simulink model "IGVC2023_LaneLines_PublishingwLabels"  (R2022a)
settings: Solver=FixedStepAuto  StartTime=0.0  StopTime=inf  RelTol=1e-3  AbsTol=1e-3
model workspace (MAT data in the model file):
  SL_ROS_VariableLengthArrays_MaxSizes.CommonInfo.ArrayTruncateAction = 'EmitWarning'
  SL_ROS_VariableLengthArrays_MaxSizes.MsgTypeMap = containers.Map
  SL_ROS_VariableLengthArrays_MaxSizes.MsgTypeMap.serialization.keys = {'sensor_msgs/Image', 'sensor_msgs/PointCloud2'}
  SL_ROS_VariableLengthArrays_MaxSizes.MsgTypeMap.serialization.values{1}(1).PropertyName = 'Data'
  SL_ROS_VariableLengthArrays_MaxSizes.MsgTypeMap.serialization.values{1}(1).DataType = 'uint8'
  SL_ROS_VariableLengthArrays_MaxSizes.MsgTypeMap.serialization.values{1}(1).MaxLength = 3686400
  SL_ROS_VariableLengthArrays_MaxSizes.MsgTypeMap.serialization.values{1}(2).PropertyName = 'Encoding'
  SL_ROS_VariableLengthArrays_MaxSizes.MsgTypeMap.serialization.values{1}(2).DataType = 'uint8'
  SL_ROS_VariableLengthArrays_MaxSizes.MsgTypeMap.serialization.values{1}(2).MaxLength = 128
  SL_ROS_VariableLengthArrays_MaxSizes.MsgTypeMap.serialization.values{2}(1).PropertyName = 'Data'
  SL_ROS_VariableLengthArrays_MaxSizes.MsgTypeMap.serialization.values{2}(1).DataType = 'uint8'
  SL_ROS_VariableLengthArrays_MaxSizes.MsgTypeMap.serialization.values{2}(1).MaxLength = 100000
  SL_ROS_VariableLengthArrays_MaxSizes.MsgTypeMap.serialization.values{2}(2).PropertyName = 'Fields'
  SL_ROS_VariableLengthArrays_MaxSizes.MsgTypeMap.serialization.values{2}(2).DataType = 'sensor_msgs/PointField'
  SL_ROS_VariableLengthArrays_MaxSizes.MsgTypeMap.serialization.values{2}(2).MaxLength = 16
  SL_ROS_VariableLengthArrays_MaxSizes.MsgTypeMap.serialization.uniformity = 0
  SL_ROS_VariableLengthArrays_MaxSizes.MsgTypeMap.serialization.keyType = 'char'
  SL_ROS_VariableLengthArrays_MaxSizes.MsgTypeMap.serialization.valueType = 'any'
undefined symbols (not defined in the file): coder, gray, ros
libraries: robotlib x42, visionconversions x2, visionmorphops x2, visiongeotforms x2, visionstatistics x1, visionsources x1
settings Model: Creator=ll  LastModifiedBy=ll
settings OptimizationCC: EnhancedBackFolding=on  PassReuseOutputArgsAs=Individual arguments  ZeroExternalMemoryAtStartup=off  ZeroInternalMemoryAtStartup=off  MaxStackSize=64  OptimizeBlockOrder=speed  DifferentSizesBufferReuse=on  OptimizationCustomize=off  EfficientTunableParamExpr=on
settings DebuggingCC: ParameterTunabilityLossMsg=error
settings HardwareCC: ProdBitPerPointer=32  ProdBitPerSizeT=32  ProdBitPerPtrDiffT=32  ProdLargestAtomicFloat=None  ProdIntDivRoundTo=Undefined  ProdEndianess=Unspecified  ProdWordSize=32  ProdHWDeviceType=Generic->Unspecified (assume 32-bit Generic)
settings RTWCC: SystemTargetFile=ert.tlc  HardwareBoard=Robot Operating System (ROS)  TLCOptions="-aInlineSetEventsForThisBaseRateFcn=TLC_FALSE -aSuppressMultiTaskScheduler=TLC_FALSE  -aRateBasedStepFcn=0"  TemplateMakefile=ert_default_tmf  Toolchain=Catkin  TargetLang=C++
settings CodeAppCC: ForceParamTrailComments=on  IgnoreCustomStorageClasses=off  OperatorAnnotations=on  SimulinkDataObjDesc=on  SFDataObjDesc=on  InsertBlockDesc=on
settings ERTTargetCC: SupportVariableSizeSignals=on

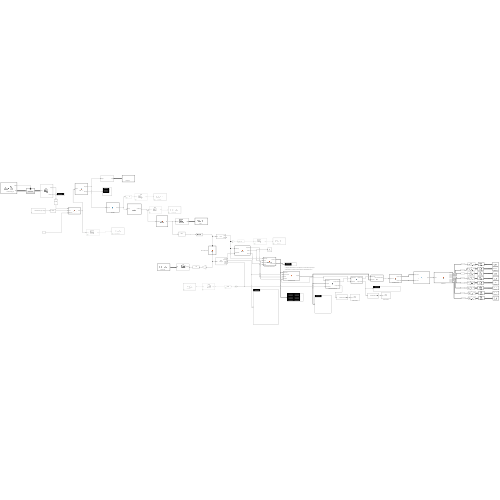
[thumbnail: Simulink's stored preview of the top-level diagram]
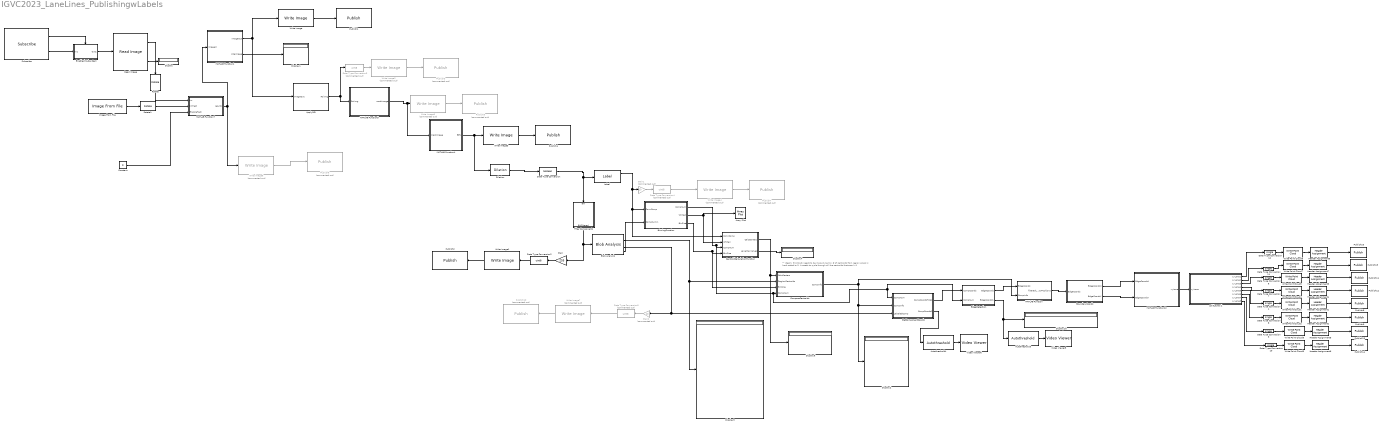
== system IGVC2023_LaneLines_PublishingwLabels ==
  note: ** ideally this block needs to be more dynamic, # of centroids from region props
      | is hard coded to 3. it needs to cycle through all the centroids that aren't -1
  ApplyROI : MATLAB Function  TreatAsAtomicUnit=on
  Array Plot : ArrayPlot  WindowPosition=[1055.000000,29.000000,800.000000,500.000000,]  ScopeFrameLocation=window  MaximizeAxes=Off
  Autothreshold3 : visionconversions/Autothreshold  operator=>  threshOut=off  effMetricOut=off  userDefinedRange=off  umin=0  umax=255  outOfRngOpt=Ignore  scaleThreshold=off  scaleFactor=1  roundingMode=Floor  overflowMode=off  P1Mode=Specify word length  P1WordLength=32  P1FracLength=30  P2Mode=Specify word length  P2WordLength=32  P2FracLength=22  P3Mode=Specify word length  P3WordLength=32  P3FracLength=14  P4Mode=Binary point scaling  P4WordLength=32  P4FracLength=15  Q1Mode=Specify word length  Q1WordLength=32  Q1FracLength=16  EMMode=Specify word length  EMWordLength=16  EMFracLength=14
      settings: SourceProductBaseCode=VP
  Autothreshold4 : visionconversions/Autothreshold  operator=>  threshOut=off  effMetricOut=off  userDefinedRange=off  umin=0  umax=255  outOfRngOpt=Ignore  scaleThreshold=off  scaleFactor=1  roundingMode=Floor  overflowMode=off  P1Mode=Specify word length  P1WordLength=32  P1FracLength=30  P2Mode=Specify word length  P2WordLength=32  P2FracLength=22  P3Mode=Specify word length  P3WordLength=32  P3FracLength=14  P4Mode=Binary point scaling  P4WordLength=32  P4FracLength=15  Q1Mode=Specify word length  Q1WordLength=32  Q1FracLength=16  EMMode=Specify word length  EMWordLength=16  EMFracLength=14
      settings: SourceProductBaseCode=VP
  BinningFunction : MATLAB Function  TreatAsAtomicUnit=on
  Blob Analysis : visionstatistics/Blob Analysis  Tag=vipblks_row_conv  area=on  centroid=on  bBox=on  majorAxis=off  minorAxis=off  angle=off  eccentricity=off  equivDiameterSq=off  extent=off  perimeter=off  outDT=double  conn=8  isLabel=on  maxBlobs=10000  warnIfNumBlobsExceeded=on  isCount=on  useMinArea=off  minArea=0  useMaxArea=off  maxArea=intmax('uint32')  excludeBorderBlob=off  isOutVarDim=off  isFill=on  fillValues=-1  roundingMode=Floor  overflowMode=off  prodOutputMode=Binary point scaling  prodOutputWordLength=32  prodOutputFracLength=16  accumMode=Binary point scaling  accumWordLength=32  accumFracLength=0  outputMode=Binary point scaling  outputWordLength=32  outputFracLength=16  firstCoeffMode=Binary point scaling  firstCoeffWordLength=16  firstCoeffFracLength=14  secondCoeffMode=Binary point scaling  secondCoeffWordLength=32  secondCoeffFracLength=16
  BoundaryCoords : MATLAB Function  TreatAsAtomicUnit=on
  CentroidCalculationFunction : MATLAB Function  TreatAsAtomicUnit=on
  CompareCentroids : MATLAB Function  TreatAsAtomicUnit=on
  Constant : Constant  Value=0
  Data Type Conversion : DataTypeConversion  OutDataTypeStr=boolean  SaturateOnIntegerOverflow=off  RndMeth=Floor
  Data Type Conversion{1,6..12} (8 alike) : DataTypeConversion  OutDataTypeStr=single  SaturateOnIntegerOverflow=off  RndMeth=Floor
  Data Type Conversion2 : DataTypeConversion  OutDataTypeStr=uint8  SaturateOnIntegerOverflow=off  RndMeth=Floor
  Data Type Conversion3 : DataTypeConversion  Commented=on  OutDataTypeStr=uint8  SaturateOnIntegerOverflow=off  RndMeth=Floor
  Data Type Conversion4 : DataTypeConversion  Commented=on  OutDataTypeStr=uint8  SaturateOnIntegerOverflow=off  RndMeth=Floor
  Data Type Conversion5 : DataTypeConversion  Commented=on  OutDataTypeStr=uint8  SaturateOnIntegerOverflow=off  RndMeth=Floor
  Dilation : visionmorphops/Dilation  nhoodsrc=Specify via dialog  strel=[1 1 1; 1 1 1; 1 1 1]
      settings: SourceProductBaseCode=VP
  Display{,1..4,6,16} (7 alike) : Display
  EdgeDetection : MATLAB Function  TreatAsAtomicUnit=on
  Enabled Subsystem : Subsystem  TreatAsAtomicUnit=on
  "Filter Components " : MATLAB Function  TreatAsAtomicUnit=on
  Gain : Gain  Gain=255
  Gain1 : Gain  Commented=on  Gain=10
  Gain2 : Gain  Commented=on  Gain=10
  GetComponentCoords : MATLAB Function  TreatAsAtomicUnit=on
  Header Assignment{1..8} (8 alike) : robotlib/Header Assignment  SetFrameID=on  FrameID=map  InsertTimeStamp=on  SetHeaderFieldName=Use the default Header field name  HeaderFieldName=Header
      settings: SourceProductBaseCode=RR
  Image From File : visionsources/Image From File  Tag=vipblks_nd  FileName=/home/ll/catkin_ws/lanesonCourse.png  Ts=inf  imagePorts=One multidimensional signal  OutPortLabels=R|G|B  ImageDataType=Inherit from input image  sdImageDataType=uint(8)  Signed=on  WordLength=16  FractionLengthMode=User-defined  FractionLength=15
  Label : visionmorphops/Label  conn=8  output=Label matrix and number of labels  outType=uint8  lastLabel=maximum value of the output data type
      settings: SourceProductBaseCode=VP
  MATLAB Function : MATLAB Function  TreatAsAtomicUnit=on
  MATLAB Function1 : MATLAB Function  TreatAsAtomicUnit=on
  MATLAB Function12 : MATLAB Function  TreatAsAtomicUnit=on
  MATLAB Function4 : MATLAB Function  TreatAsAtomicUnit=on
  MATLAB Function5 : MATLAB Function  TreatAsAtomicUnit=on
  MATLAB Function7 : MATLAB Function  TreatAsAtomicUnit=on
  Publish1 : robotlib/Publish  topicSource=Specify your own  topic=/grayimage  messageType=sensor_msgs/Image  legacyBusStruct=off  messageQueueLength=1
  Publish10 : robotlib/Publish  Commented=on  topicSource=Specify your own  topic=/Labeled1  messageType=sensor_msgs/Image  legacyBusStruct=off  messageQueueLength=1
  Publish11 : robotlib/Publish  topicSource=Specify your own  topic=/lanes3  messageType=sensor_msgs/PointCloud2  legacyBusStruct=off  messageQueueLength=1
  Publish12 : robotlib/Publish  topicSource=Specify your own  topic=/lanes4  messageType=sensor_msgs/PointCloud2  legacyBusStruct=off  messageQueueLength=1
  Publish13 : robotlib/Publish  topicSource=Specify your own  topic=/lanes7  messageType=sensor_msgs/PointCloud2  legacyBusStruct=off  messageQueueLength=1
  Publish14 : robotlib/Publish  topicSource=Specify your own  topic=/lanes8  messageType=sensor_msgs/PointCloud2  legacyBusStruct=off  messageQueueLength=1
  Publish15 : robotlib/Publish  topicSource=Specify your own  topic=/lanes2  messageType=sensor_msgs/PointCloud2  legacyBusStruct=off  messageQueueLength=1
  Publish16 : robotlib/Publish  topicSource=Specify your own  topic=/lanes1  messageType=sensor_msgs/PointCloud2  legacyBusStruct=off  messageQueueLength=1
  Publish2 : robotlib/Publish  topicSource=Specify your own  topic=/ConnComp  messageType=sensor_msgs/Image  legacyBusStruct=off  messageQueueLength=1
  Publish3 : robotlib/Publish  Commented=on  topicSource=Specify your own  topic=/rectangle  messageType=sensor_msgs/Image  legacyBusStruct=off  messageQueueLength=1
  Publish4 : robotlib/Publish  topicSource=Specify your own  topic=/BEV  messageType=sensor_msgs/Image  legacyBusStruct=off  messageQueueLength=1
  Publish5 : robotlib/Publish  Commented=on  topicSource=Specify your own  topic=/whiteimage  messageType=sensor_msgs/Image  legacyBusStruct=off  messageQueueLength=1
  Publish6 : robotlib/Publish  Commented=on  topicSource=Specify your own  topic=/originalImage  messageType=sensor_msgs/Image  legacyBusStruct=off  messageQueueLength=1
  Publish7 : robotlib/Publish  Commented=on  topicSource=Specify your own  topic=/Labeled  messageType=sensor_msgs/Image  legacyBusStruct=off  messageQueueLength=1
  Publish8 : robotlib/Publish  topicSource=Specify your own  topic=/lanes5  messageType=sensor_msgs/PointCloud2  legacyBusStruct=off  messageQueueLength=1
  Publish9 : robotlib/Publish  topicSource=Specify your own  topic=/lanes6  messageType=sensor_msgs/PointCloud2  legacyBusStruct=off  messageQueueLength=1
  Read Image : robotlib/Read Image  MaximumImageSize=[960, 1280]  ImageEncoding=bgr8  ShowAlphaOutput=off  ShowErrorCodeOutput=on  VariableSizeOutputs=off
      settings: SourceProductBaseCode=RR
  Rotate : visiongeotforms/Rotate  outSizeR=Expanded to fit rotated input image  src_angle=Specify via dialog  unit_angle=Degrees  angle=pi  maxAngle=pi  dispImage=Top-left corner  method=Table lookup  fillVal=0  interpMethod=Bilinear  roundingMode=Nearest  overflowMode=on  prodOutputMode=Binary point scaling  prodOutputWordLength=32  prodOutputFracLength=10
  Rotate1 : visiongeotforms/Rotate  outSizeR=Expanded to fit rotated input image  src_angle=Specify via dialog  unit_angle=Degrees  angle=pi  maxAngle=pi  dispImage=Top-left corner  method=Table lookup  fillVal=0  interpMethod=Bilinear  roundingMode=Nearest  overflowMode=on  prodOutputMode=Binary point scaling  prodOutputWordLength=32  prodOutputFracLength=10
  Subscribe : robotlib/Subscribe  topicSource=Select from ROS network  topic=/camera/image_raw  messageType=sensor_msgs/Image  SampleTime=-1  legacyBusStruct=off  messageQueueLength=1
  Video Viewer5 : VideoViewer  colormapValue=gray(256)  FigPos=[282 997 791 549]
  Video Viewer6 : VideoViewer  colormapValue=gray(256)  FigPos=[1110 1011 811 535]
  Write Image : robotlib/Write Image  ImageEncoding=mono8  EncodingStruct=ros.msg.sensor_msgs.internal.ImageEncoding.info(coder.const('mono8'))  HasAlpha=off  messageType=sensor_msgs/Image
      settings: SourceProductBaseCode=RR
  Write Image1 : robotlib/Write Image  ImageEncoding=mono8  EncodingStruct=ros.msg.sensor_msgs.internal.ImageEncoding.info(coder.const('mono8'))  HasAlpha=off  messageType=sensor_msgs/Image
      settings: SourceProductBaseCode=RR
  Write Image{2,4..5,7} (4 alike) : robotlib/Write Image  Commented=on  ImageEncoding=mono8  EncodingStruct=ros.msg.sensor_msgs.internal.ImageEncoding.info(coder.const('mono8'))  HasAlpha=off  messageType=sensor_msgs/Image
      settings: SourceProductBaseCode=RR
  Write Image3 : robotlib/Write Image  ImageEncoding=mono8  EncodingStruct=ros.msg.sensor_msgs.internal.ImageEncoding.info(coder.const('mono8'))  HasAlpha=off  messageType=sensor_msgs/Image
      settings: SourceProductBaseCode=RR
  Write Image6 : robotlib/Write Image  Commented=on  ImageEncoding=bgr8  EncodingStruct=ros.msg.sensor_msgs.internal.ImageEncoding.info(coder.const('bgr8'))  HasAlpha=off  messageType=sensor_msgs/Image
      settings: SourceProductBaseCode=RR
  Write Point Cloud{1..8} (8 alike) : robotlib/Write Point Cloud  Encoding=none  HasRGB=false  HasAlpha=false  FieldNamesStruct=struct('x', 'single', 'y', 'single', 'z', 'single')  messageType=sensor_msgs/PointCloud2
      settings: SourceProductBaseCode=RR
  splitLayers 1 : MATLAB Function  TreatAsAtomicUnit=on
  wires:
  Enabled Subsystem/1(Out1) -> Read Image/1
  MATLAB Function5/1(maskImage) -> MATLAB Function4/1(maskImage), Write Image5/1
  MATLAB Function1/1(ImageOut) -> Write Image/1, ApplyROI/1(ImageOut)
  MATLAB Function4/1(BEV) -> Dilation/1, Write Image3/1
  Write Image3/1 -> Publish4/1
  Subscribe/2 -> Enabled Subsystem/1(In1)
  Subscribe/1 -> Enabled Subsystem/Enable
  Write Image/1 -> Publish1/1
  Read Image/2 -> Display/1
  MATLAB Function1/2(sizeImage) -> Display1/1
  Write Image5/1 -> Publish5/1
  Label/1 -> CentroidCalculationFunction/1(ConnComp), BinningFunction/1(ConnComp), Gain1/1
  Data Type Conversion/1 -> Label/1, "Filter Components "/1(BW)
  Dilation/1 -> Data Type Conversion/1
  Constant/1 -> MATLAB Function7/3(EnableTest)
  Image From File/1 -> Rotate1/1
  Read Image/1 -> Rotate/1
  MATLAB Function7/1(results) -> Write Image6/1, MATLAB Function1/1(ImageIn)
  BinningFunction/1(CompNum) -> EdgeDetection/2(CompNum), GetComponentCoords/1(CompNum), CompareCentroids/4(CompNum), CentroidCalculationFunction/3(CompNum)
  BinningFunction/3(BinSize) -> CompareCentroids/3(BinSize), CentroidCalculationFunction/4(BinSize)
  Blob Analysis/2 -> Display3/1, CompareCentroids/2(RegionCentroids)
  CentroidCalculationFunction/1(CalcCenters) -> Display6/1, CompareCentroids/1(CalcCenters)
  CompareCentroids/1(CompInfo) -> Display2/1, GetComponentCoords/2(CompInfo), MATLAB Function/2(CompInfo)
  ApplyROI/1(RoiImg) -> Data Type Conversion3/1, MATLAB Function5/1(RoiImg)
  Write Image2/1 -> Publish3/1
  Data Type Conversion3/1 -> Write Image2/1
  Write Image1/1 -> Publish2/1
  Data Type Conversion2/1 -> Write Image1/1
  Gain/1 -> Data Type Conversion2/1
  Write Image4/1 -> Publish7/1
  Data Type Conversion4/1 -> Write Image4/1
  Gain1/1 -> Data Type Conversion4/1
  Write Image6/1 -> Publish6/1
  Rotate/1 -> MATLAB Function7/1(im)
  Rotate1/1 -> MATLAB Function7/2(imTest)
  BinningFunction/2(WhiteX) -> Array Plot/1, CentroidCalculationFunction/2(WhiteX)
  Data Type Conversion5/1 -> Write Image7/1
  Gain2/1 -> Data Type Conversion5/1
  Write Image7/1 -> Publish10/1
  Blob Analysis/5 -> BinningFunction/2(CompNumIn)
  "Filter Components "/1(BWfiltered) -> Blob Analysis/1, Gain/1
  Blob Analysis/4 -> Gain2/1, GetComponentCoords/3(LabeledComp)
  GetComponentCoords/1(CompCoordsTotal) -> EdgeDetection/1(CompCoords)
  EdgeDetection/1(EdgeCoords) -> MATLAB Function/1(EdgeCoords)
  BoundaryCoords/1(EdgeCoordsX) -> MATLAB Function12/1(EdgeCoordsX)
  BoundaryCoords/2(EdgeCoordsY) -> MATLAB Function12/2(EdgeCoordsY)
  MATLAB Function12/1(xyLane) -> splitLayers 1/1(xyLane)
  Write Point Cloud3/1 -> Header Assignment3/1
  Header Assignment3/1 -> Publish11/1
  splitLayers 1/3(xyLane3) -> Data Type Conversion6/1
  Autothreshold3/1 -> Video Viewer5/1
  EdgeDetection/2(EdgeCoords1) -> Display16/1, Autothreshold3/1
  GetComponentCoords/2(CompCoords1) -> Autothreshold4/1
  Autothreshold4/1 -> Video Viewer6/1
  Data Type Conversion6/1 -> Write Point Cloud3/1
  splitLayers 1/4(xyLane4) -> Data Type Conversion7/1
  Data Type Conversion7/1 -> Write Point Cloud4/1
  Header Assignment4/1 -> Publish12/1
  Write Point Cloud4/1 -> Header Assignment4/1
  Data Type Conversion1/1 -> Write Point Cloud1/1
  Write Point Cloud1/1 -> Header Assignment1/1
  Header Assignment1/1 -> Publish8/1
  Header Assignment2/1 -> Publish9/1
  Write Point Cloud2/1 -> Header Assignment2/1
  Data Type Conversion8/1 -> Write Point Cloud2/1
  Data Type Conversion9/1 -> Write Point Cloud5/1
  Write Point Cloud5/1 -> Header Assignment5/1
  Header Assignment5/1 -> Publish13/1
  Header Assignment6/1 -> Publish14/1
  Write Point Cloud6/1 -> Header Assignment6/1
  Data Type Conversion10/1 -> Write Point Cloud6/1
  Data Type Conversion11/1 -> Write Point Cloud7/1
  Write Point Cloud7/1 -> Header Assignment7/1
  Header Assignment7/1 -> Publish15/1
  Data Type Conversion12/1 -> Write Point Cloud8/1
  Write Point Cloud8/1 -> Header Assignment8/1
  Header Assignment8/1 -> Publish16/1
  splitLayers 1/1(xyLane1) -> Data Type Conversion12/1
  splitLayers 1/2(xyLane2) -> Data Type Conversion11/1
  splitLayers 1/5(xyLane5) -> Data Type Conversion1/1
  splitLayers 1/6(xyLane6) -> Data Type Conversion8/1
  splitLayers 1/7(xyLane7) -> Data Type Conversion9/1
  splitLayers 1/8(xyLane8) -> Data Type Conversion10/1
  MATLAB Function/1(filteredLaneswPositions) -> BoundaryCoords/1(EdgeCoords)
  CentroidCalculationFunction/2(LaneMaxValues) -> Display4/1

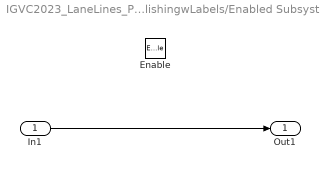
== system IGVC2023_LaneLines_PublishingwLabels/Enabled Subsystem ==
  In1 : Inport
  Enable : EnablePort
  Out1 : Outport
  wires:
  In1/1 -> Out1/1

== matlab function IGVC2023_LaneLines_PublishingwLabels/GetComponentCoords ==
  data: CompNum input; CompInfo input; LabeledComp input; CompCoordsTotal output; CompCoords1 output
function [CompCoordsTotal,CompCoords1]= fcn(  CompNum, CompInfo, LabeledComp)

PointNum = single(1500);

[InfoX, ~] = size(CompInfo);
CompCoords = zeros(2500,1280,8);
CompCoords1 = zeros(2500, 1280);
CompCoordsTotal= zeros(2500, 1280,8);
BoundaryCoords = uint16(zeros(50000, 2,8));
EditedBoundaryCoords = uint16(zeros(5000, 2,8));
BoundaryCoords1 = uint16(zeros(5000, 2,1));
labelMarix = zeros(2500);
 CompR = 0;
 CompC = 0;
 lastPoint=zeros(1,2);
 step = 100;
 x=0;y=0;yPoint=0;
 CompCSize =0;
 CompRSize =0;
 emptyStat = "true";
 Unused = [0 0];

 [sizeX,~]=size(CompInfo);
if sizeX > 8
    sizeX =8;
end
for i=1:sizeX

%for i = 1:CompNum
 ymin = 1;
 ymax = 1;
 xmin = 1;
 xmax = 1; 

    if CompInfo(i, 2) == 1
    
        windowWidth =40;
        windowStart = round(CompInfo(i,1) - (windowWidth/2));
        windowEnd = round(CompInfo(i,1) + (windowWidth/2));
        LabelOfComponents=unique(LabeledComp(:,round(CompInfo(i,1))));
    
        LabelOfComponents(LabelOfComponents==0)=[];
        [numOfCompinLane,~]=size(LabelOfComponents);
        CompCoordsTotal(:,:,i)=0;
for k=1:numOfCompinLane
       CompCoords(:,:,i) = (LabeledComp == LabelOfComponents(k));
       CompCoordsTotal(:,:,i) = CompCoordsTotal(:,:,i) + CompCoords(:,:,i);
%LabelOfComponents = unique(LabeledComp(:,round(CompInfo(i,1))))
       % [NumberofComponentsinLane, ~] = size(LabelOfComponents);

    end
    end
    CompCoords1(:,:) = CompCoordsTotal(:,:,3);
end

== matlab function IGVC2023_LaneLines_PublishingwLabels/EdgeDetection ==
  data: CompCoords input; EdgeCoords output; CompNum input; EdgeCoords1 output
function [EdgeCoords,EdgeCoords1]= fcn(CompCoords, CompNum)

EdgeCoords = zeros(2500,1280,8);
EdgeCoords1 = zeros(2500,1280);

for i=1:8
EdgeCoords(:,:,i)=edge(CompCoords(:,:,i),'sobel');
end
EdgeCoords1=EdgeCoords(:,:,3);
end

== matlab function IGVC2023_LaneLines_PublishingwLabels/BoundaryCoords ==
  data: EdgeCoordsX output size=[8000 1 8]; EdgeCoords input; EdgeCoordsY output size=[8000 1 8]
function [EdgeCoordsX,EdgeCoordsY]= fcn(EdgeCoords)

EdgeCoordsX=zeros(8000,1,8);
EdgeCoordsX1=zeros(5500,1,1);
Indices=zeros(5000,1,8);
EdgeCoordsY=zeros(8000,1,8);
Index1=zeros(5000);
img = zeros(2500,1280);

for i=1:8
    if nnz(EdgeCoords(:,:,i)) >=1
        addLimit = nnz(EdgeCoords(:,:,i));
[EdgeCoordsY(1:addLimit,:,i), EdgeCoordsX(1:addLimit,:,i)] = find(EdgeCoords(:,:,i) == 1);
%Indices(1:addLimit,:,i) = find(EdgeCoords(:,:,i) == 1);
    end
end
%EdgeCoordsX1(:,:) = EdgeCoordsX(:,:,3);
%img(Indices(:,:,4))=1;
end

== matlab function IGVC2023_LaneLines_PublishingwLabels/MATLAB Function12 ==
  data: xyLane output size=[8000 2 8]; EdgeCoordsX input; EdgeCoordsY input
function xyLane  = image2distance(EdgeCoordsX, EdgeCoordsY)
%#codegen

%xyimageLeft(1,:)=xyimageLeft(1,:);
%xyimageRight(1,:)=xyimageRight(1,:);
5500
%Transform Road Image to Bird's-Eye-View Image
%Create a bird's-eye-view image from an image obtained by a front-facing camera mounted on a vehicle. Display points within the bird's-eye view using the vehicle and image coordinate systems.
%Define the camera intrinsics and create an object containing these intrinsics.
%focalLength = [309.4362 344.2161];
%focalLength=[274.769879268627	124.585825090253];
%focalLength=[950.730389523017	872.418095589972];
%249.386359893401	113.313356588451
%principalPoint = [318.9034 257.5352];
%principalPoint = [618.652151593579	622.123926433697];
%principalPoint = [666.407201481039	199.198016715410];
%617.370454615737	627.572919668628

%copied from workspace
focalLength=[1.036287558959034e+03,1.056617977212135e+03];
principalPoint=[5.907584934807890e+02,4.225814969478901e+02];

%imageSize = [480 640];
imageSize = [2500	1280];
%datasize=size(xyimageLeft);

camIntrinsics = cameraIntrinsics(focalLength,principalPoint,imageSize);

%Set the height of the camera to be about 2 meters above the ground. Set the pitch of the camera to 14 degrees toward the ground.
 height = 1.524; %in meters
 pitch = 8.5;
% 
%Create an object containing the camera configuration.
sensor = monoCamera(camIntrinsics,height,'Pitch',pitch);

% %Define the area in front of the camera that you want to transform into a bird's-eye view. Set an area from 3 to 30 meters in front of the camera, with 6 meters to either side of the camera.
distAhead = 10; %originally 5
spaceToOneSide = 6;
bottomOffset = 1;
outView = [bottomOffset,distAhead,-spaceToOneSide,spaceToOneSide];

%Set the output image width to 250 pixels. Compute the output length automatically from the width by setting the length to NaN.
%outImageSize = [1024,250];
outImageSize = [2879,1280];

xyForm=zeros(8000,2);
%Create an object for performing bird's-eye-view transforms, using the previously defined parameters.
birdsEye = birdsEyeView(sensor,outView,outImageSize);
%xyL=[xyimageLeft(1,:)'*dwidth,xyimageLeft(1,:)'*dheight];%
%xyL=imageToVehicle(birdsEye,xyimageLeft');
%xyR=[xyimageRight(1,:)'*dwidth,xyimageRight(1,:)'*dheight];%
%xyR=imageToVehicle(birdsEye,xyimageRight');
xyLane=zeros(8000,2,8);
%xyvehicle=zeros(3000,2,8);
%thisComponent = zeros(PointNum,2,8); 

for k=1:8
%thisComponent = single(EditedboundaryCoords(:,:,k));
%xySize = numel(EditedboundaryCoords(:,1,k));
xyForm(:,1)= EdgeCoordsX(:,:,k);
xyForm(:,2)= EdgeCoordsY(:,:,k);
xyLane(:,:,k)=imageToVehicle(birdsEye,xyForm);
%laneZeros = zeros(length(xyLane),1,k);
%xyvehicle(:,:,k)= single([xyLane(:,:,k),laneZeros]);
end
%xyvehicleleft = single([xyL,zeros(length(xyL),1)]);
%xyvehicleright= single([xyR,zeros(length(xyR),1)]);
%datasizeL=size(xyvehicleleft);
%datasizeR=size(xyvehicleright);
%datasize=size(xyvehicle);

== matlab function IGVC2023_LaneLines_PublishingwLabels/splitLayers 1 ==
  data: xyLane input; xyLane1 output size=[8000 3 1]; xyLane2 output size=[8000 3 1]; xyLane3 output size=[8000 3 1]; xyLane4 output size=[8000 3 1]; xyLane5 output size=[8000 3 1]; xyLane6 output size=[8000 3 1]; xyLane7 output size=[8000 3 1]; xyLane8 output size=[8000 3 1]
function [xyLane1,xyLane2,xyLane3,xyLane4,xyLane5,xyLane6,xyLane7,xyLane8]= fcn(xyLane)

laneStatus = "No Status" ;
xyLane1 = zeros(8000, 3);
xyLane2 = zeros(8000, 3);
xyLane3 = zeros(8000, 3);
xyLane4 = zeros(8000, 3);
xyLane5 = zeros(8000, 3);
xyLane6 = zeros(8000, 3);
xyLane7 = zeros(8000, 3);
xyLane8 = zeros(8000, 3);

[Xlength, Ylength, Zlength] = size(xyLane);

if Zlength > 8 
    laneStatus = "Z size fault, more than 8 objects";
end

if Zlength <= 8
    for i=1:8
        switch i
            case 1
                    %xyLane1 = xyLane(:,1:2,1);
                    %laneZeros = zeros(length(xyLane1));
                    xyLane1 = ([xyLane(:,:,1),zeros(length(xyLane),1)]);
                  % 
            case 2
                    %xyLane2 = xyLane(:,1:2,2);
                    xyLane2 = ([xyLane(:,:,2),zeros(length(xyLane),1)]);
            case 3
                  %  xyLane3 = xyLane(:,1:2,3);
                    xyLane3 = ([xyLane(:,:,3),zeros(length(xyLane),1)]);
                
            case 4
                   % xyLane4 = xyLane(:,:,4);
                    xyLane4 = ([xyLane(:,:,4),zeros(length(xyLane),1)]);
            case 5
                    %xyLane5 = xyLane(:,:,5);
                    xyLane5 = ([xyLane(:,:,5),zeros(length(xyLane),1)]);
                
            case 6
                    %xyLane6 = xyLane(:,:,6);
                    xyLane6 = ([xyLane(:,:,6),zeros(length(xyLane),1)]);
                
            case 7
                    %xyLane7 = xyLane(:,:,7);
                    xyLane7 = ([xyLane(:,:,7),zeros(length(xyLane),1)]);
                
            case 8
                    %xyLane8 = xyLane(:,:,8);
                    xyLane8 = ([xyLane(:,:,8),zeros(length(xyLane),1)]);
         end 
    end
end

y=1;

== matlab function IGVC2023_LaneLines_PublishingwLabels/MATLAB Function1 ==
  data: ImageIn input; ImageOut output; sizeImage output
function [ImageOut,sizeImage]= grayImage(ImageIn)

sizeImage=size(ImageIn);

ImageOut=im2uint8(im2gray(ImageIn));
%ImageOut= uint8(imbinarize(GrayImg, 'adaptive', 'Sensitivity', 0.500000, 'ForegroundPolarity', 'bright'));

== matlab function IGVC2023_LaneLines_PublishingwLabels/MATLAB Function4 ==
  data: maskImage input; BEV output
function BEV = BEVimage(maskImage)
%Transform Road Image to Bird's-Eye-View Image
%Create a bird's-eye-view image from an image obtained by a front-facing 
% camera mounted on a vehicle. Display points within the bird's-eye view 
% using the vehicle and image coordinate systems.
%Define the camera intrinsics and create an object containing these intrinsics.
%focalLength = [309.4362 344.2161];
%focalLength=[274.769879268627	124.585825090253];
%focalLength=[9.485122935354788e+02,9.419404214092846e+02];
%249.386359893401	113.313356588451
%principalPoint = [318.9034 257.5352];
%principalPoint = [618.652151593579	622.123926433697];
%principalPoint = [5.819667727643726e+02,4.692273010971225e+02];
%617.370454615737	627.572919668628
focalLength=[1.036287558959034e+03,1.056617977212135e+03];
principalPoint=[5.907584934807890e+02,4.225814969478901e+02];
%imageSize = [480 640];
imageSize = [960	1280];

%datasize=size(xyimageLeft);

camIntrinsics = cameraIntrinsics(focalLength,principalPoint,imageSize);

%Set the height of the camera to be about 2 meters above the ground. 
% Set the pitch of the camera to 14 degrees toward the ground.
 height = 1.524; %in meters
 pitch = 8.5;
% 
%Create an object containing the camera configuration.
sensor = monoCamera(camIntrinsics,height,'Pitch',pitch);
% 
% %Define the area in front of the camera that you want to transform into 
% a bird's-eye view. Set an area from 3 to 30 meters in front of the camera, 
% with 6 meters to either side of the camera.
distAhead = 7;
spaceToOneSide = 6;
bottomOffset = 0.5;
outView = [bottomOffset,distAhead,-spaceToOneSide,spaceToOneSide];

%Set the output image width to 250 pixels. Compute the output length 
% automatically from the width by setting the length to NaN.
outImageSize = [2500 1280];
%Create an object for performing bird's-eye-view transforms, using the 
% previously defined parameters.
birdsEye = birdsEyeView(sensor,outView,outImageSize);

BEV1 = transformImage(birdsEye,maskImage);
BEV = imresize(BEV1,[2500 1280]);

== matlab function IGVC2023_LaneLines_PublishingwLabels/MATLAB Function ==
  data: EdgeCoords input; filteredLaneswPositions output; CompInfo input
function filteredLaneswPositions = fcn(EdgeCoords, CompInfo)

laneSplit = 1280/2;
%laneSplit = 5;
compNum = 4;

filteredLaneswPositions = zeros(2500,1280,8);
[sizeX,~]=size(CompInfo);
if sizeX > 8
    sizeX =8;
end
for m=1:sizeX

   if CompInfo(m,1) > laneSplit && CompInfo(m,2)==1 && sum(filteredLaneswPositions(:,:,5),"all")==0 %greater than lane split therefore left lane
       filteredLaneswPositions(:,:,5) = EdgeCoords(:,:,m);        
   elseif CompInfo(m,1) > laneSplit && CompInfo(m,2)==1 && sum(filteredLaneswPositions(:,:,5),"all")>0  && sum(filteredLaneswPositions(:,:,6),"all")==0 %greater than lane split and 3 full so left adjecent lane
       filteredLaneswPositions(:,:,6) = EdgeCoords(:,:,m); 
   elseif CompInfo(m,1) < laneSplit && CompInfo(m,2)==1 && sum(filteredLaneswPositions(:,:,4),"all")==0 %less than so right lane
       filteredLaneswPositions(:,:,4) = EdgeCoords(:,:,m); 
   elseif CompInfo(m,1) < laneSplit && CompInfo(m,2)==1 && sum(filteredLaneswPositions(:,:,4),"all")>0  && sum(filteredLaneswPositions(:,:,3),"all")==0 %less than and 2 filled so right adjecent lane
       filteredLaneswPositions(:,:,3) = EdgeCoords(:,:,m);
   end
end

== matlab function IGVC2023_LaneLines_PublishingwLabels/MATLAB Function5 ==
  data: RoiImg input; maskImage output
function maskImage = whiteMask(RoiImg) 
maskImage1 = zeros(size(RoiImg,1),size(RoiImg,2));

% %----------------------Define thresholds for 'Hue'---------------------
 %channel1MinW = 200;
 %channel1MaxW = 255;
% %------------------Define thresholds for 'Saturation'------------------
% channel2MinW = 200;
% channel2MaxW = 255;
% %---------------------Define thresholds for 'Value'--------------------
% channel3MinW = 200;
% channel3MaxW = 255;

%-----------Create mask based on chosen histogram thresholds-----------

for i = 1:size(RoiImg,1)
    for j = 1:size(RoiImg,2)
        if ((RoiImg(i,j)>=200))
            maskImage1(i,j)  = 255;
        end
    end
end

maskImage = im2uint8(maskImage1);
 %maskImage=(ImageOut(:,:)>=channel1MinW)|(ImageOut(:,:)<=channel1MaxW);


%maskImage = imresize(maskImage1, [600 1280]);

== matlab function IGVC2023_LaneLines_PublishingwLabels/BinningFunction ==
  data: ConnComp input; CompNum output; CompNumIn input; WhiteX output; BinSize output
function [CompNum,WhiteX,BinSize] = Binning(ConnComp,CompNumIn)

CompNum=uint16(CompNumIn);

%CompProps = struct;
%CompNum = max(CompLabels,[],'all','linear');

%CompProps = regionprops(ConnComp, 'All');
%ERROR: accessing field or property of nonscalar struct or object not supported
%for code generation in this context
%the following is a work around from https://stackoverflow.com/questions/72298202/how-to-solve-directly-accessing-field-or-property-of-nonscalar-struct-or-object
%PropNums = numel(CompProps);
%centroidPoints = coder.nullcopy(zeros(PropNums,2, "double"));
%for idx = 1:PropNums
%    centroidPoints(idx,1) = double(CompProps(idx).Centroid(1));
%end

%allCompCentroids = vertcat(CompProps.Centroid);% A 10 row by 2 column array of (x,y) centroid coordinates.
%centroidsX = allCompCentroids(:, 1);% Extract out the centroid x values into their own vector.
%centroidsY = allCompCentroids(:, 2);

%BinNum = 100;
BinSize = 10;
BinNum = 128;
BinStart=1;
Bin = 1;
WhiteX = zeros(BinNum,1);
%A=zeros(10,1);
%BinEndMinus1 = 
BinEnd=9;
for BinEnd=9:BinSize:1280 
  sumV=0;
    for inc=BinStart:1:BinEnd
        sumV=sum(ConnComp(:,inc))+sumV;
    end

    WhiteX(Bin,1) = sumV;%sum(ConnComp(:,A));
    Bin = Bin+1;
    BinStart=BinEnd+1;
end

%plot(WhiteX(:,:))
%axis([0 BinNum 0 max(WhiteX)])
%find local maximums because each peak has mulitple points so just maxs
%wont work

%MinProm = 500;
% LocalMaxima = islocalmax(WhiteX, "MinProminence",MinProm);
%LocalMaxima = imregionalmax(WhiteX);
%[maximaR, maximaC] = find(LocalMaxima==1);
% LocalMaxValues=zeros(CompNum,2);
% LaneMaxR=zeros(CompNum,2);
% LaneMaxC=zeros(CompNum,2);
% %now that we have local max index, we compare to whiteX to get value and then we grab the two maxes from there.
% for k=1:1:numel(maximaR)
% LocalMaxValues(k,1) = WhiteX(maximaR(k),1);
% end
% 
% LaneMaxValues = maxk(LocalMaxValues,2);
% [LaneMaxR(1), LaneMaxC(1)] = find(WhiteX==LaneMaxValues(1));
% [LaneMaxR(2), LaneMaxC(2)] = find(WhiteX==LaneMaxValues(2));
% %convert back to coord
% CalcCenters = LaneMaxR(:)*BinSize;
% 
% 
% %Comparing cetroids to white graph maxima to check if what we have are lane lines
% WhitePtTolerance = BinSize + 7; %adding a little bit of extra tolerance because these aren't in bird's eye
% CompInfo = zeros(CompNum, 2);
% for i = 1:1:CompNum
%     CompInfo (i,1) = centroidPoints(i,1);
%     CompInfo(i,2) = 0; %initalize to prevet false pos
%     CentroidDifference1 = abs(CalcCenters(1)-centroidPoints(i,1));
%     CentroidDifference2 = abs(CalcCenters(2)-centroidPoints(i,2));
% 
%     if (CentroidDifference1 <= WhitePtTolerance || CentroidDifference2 <= WhitePtTolerance)
%         CompInfo(i,2) = 1; %true does match
%     end
% end
% 
%     %coder.varsize('CompBoundries',[960 1280], [1 0]);
% for k = 1 : CompNum           % Loop through all comp.
%     % Place the comp label number at the centroid of the blob.
%     if(CompInfo(k,2)==1)
% %text(centroidsX(k), centroidsY(k), num2str(k), 'FontSize', 14, 'FontWeight', 'Bold', 'HorizontalAlignment', 'center', 'VerticalAlignment', 'middle');
%     CompBoundries = bwboundaries(ConnComp,8,'noholes');
%     hold on;
%     thisBoundary = CompBoundries{k}; % Get boundary for this component
% 
%     InitBoundaryCoords(:,1,k) = thisBoundary(:,1);
%     InitBoundaryCoords(:,2,k) = thisBoundary(:,2);
%     % Column 2 is the columns, which is x % Column 1 is the rows, which is y
%     %plot(x, y, 'r-', 'LineWidth', 3.5); % Plot boundary in red.
%     end
% end

%boundaryCoords=InitBoundaryCoords;

== matlab function IGVC2023_LaneLines_PublishingwLabels/CentroidCalculationFunction ==
  data: ConnComp input; CalcCenters output size=10000 [1..10000]; WhiteX input; CompNum input; BinSize input; LaneMaxValues output size=5
function [CalcCenters,LaneMaxValues]= FindCentroid(ConnComp,WhiteX,CompNum, BinSize)

%find local maximums because each peak has mulitple points so just maxs
%wont work

MinProm = 300;
LocalMaxima = zeros(CompNum, 1);
LocalMaxima = double(islocalmax(WhiteX, "MinProminence",MinProm));
%maximaCoords = zeros(10000,1);
[maximaCoords]= single(abs(find(LocalMaxima==1,CompNum)));

%[maximaR, maximaC] = find(LocalMaxima==1);
LocalMaxValues=zeros(CompNum,1);
LaneMaxR=zeros(CompNum,2);
LaneMaxC=zeros(CompNum,2);
%now that we have local max index, we compare to whiteX to get value and then we grab the two maxes from there.
for k=1:1:numel(maximaCoords)
    LocalMaxValues(k) = WhiteX(maximaCoords(k),1);
end

LaneMaxValues = maxk(LocalMaxValues,2);
if sum(LaneMaxValues(1),"all")>0
[LaneMaxR(1), ~] = find(WhiteX==LaneMaxValues(1));
end
if size(LaneMaxValues)>1
[LaneMaxR(2), ~] = find(WhiteX==LaneMaxValues(2));
% %convert back to(2,:),"all" coordrenameutils
end
CalcCenters = LaneMaxR(:)*BinSize;
% 
% 
% %Comparing cetroids to white graph maxima to check if what we have are lane lines
% WhitePtTolerance = BinSize + 7; %adding a little bit of extra tolerance because these aren't in bird's eye
% CompInfo = zeros(CompNum, 2);
% for i = 1:1:CompNum8000800080008000
%     CompInfo (i,1) = centroidPoints(i,LaneMaxValues1);
%     CompInfo(i,2) = 0; %initalize to prevet false pos
%     CentroidDifference1 = abs(CalcCenters(1)-centroidPoints(i,1));80008000
%     CentroidDifference2 = abs(CalcCenters(2)-centroidPoints(i,2));
% 
%     if (CentroidDifference1 <= WhitePtTolerance || CentroidDifference2 <= WhitePtTolerance)
%         CompInfo(i,2) = 1; %true does match
%     end
% end
% 
%     %coder.varsize('CompBoundries',[960 1280], [1 0]);
% for k = 1 : CompNum           % Loop through all comp.
%     % Place the comp label number at the centroid of the blob.
%     if(CompInfo(k,2)==1)
% %text(centroidsX(k), centroidsY(k), num2str(k), 'FontSize', 14, 'FontWeight', 'Bold', 'HorizontalAlignment', 'center', 'VerticalAlignment', 'middle');
%     CompBoundries = bwboundaries(ConnComp,8,'noholes');
%     hold on;
%     thisBoundary = CompBoundries{k}; % Get boundary for this component
% 
%     InitBoundaryCoords(:,1,k) = thisBoundary(:,1);
%     InitBoundaryCoords(:,2,k) = thisBoundary(:,2);
%     % Column 2 is the columns, which is x % Column 1 is the rows, which is y
%     %plot(x, y, 'r-', 'LineWidth', 3.5); % Plot boundary in red.
%     end
% end

== matlab function IGVC2023_LaneLines_PublishingwLabels/CompareCentroids ==
  data: CalcCenters input; RegionCentroids input; CompInfo output size=[1000 2]; BinSize input; CompNum input
function CompInfo = fcn(CalcCenters, RegionCentroids, BinSize, CompNum)

%Comparing cetroids to white graph maxima to check if what we have are lane lines
WhitePtTolerance = BinSize + 5; 
CompInfo = zeros(CompNum, 2);
[sizeX,sizeY]=size(CompInfo)
for i = 1:1:CompNum 
    CentroidDifference1 = 0;
    CentroidDifference2 = 0;
    [centroidNum,centroidSize] = size(RegionCentroids)
    %for j = 1:centroidNum
    %CompInfo(i,2) = 0; %initalize/reset this
    CompInfo (i,1) = RegionCentroids(i,1);
    CompInfo(i,2) = 0; %initalize to prevet false pos
    CentroidDifference1 = abs(RegionCentroids(i,1)-CalcCenters(1))
    CentroidDifference2 = abs(RegionCentroids(i,1)-CalcCenters(2))

    if (CentroidDifference1 <= WhitePtTolerance || CentroidDifference2 <= WhitePtTolerance)
        CompInfo(i,2) = 1; %true does match
    elseif (CentroidDifference1 > WhitePtTolerance && CentroidDifference2 > WhitePtTolerance)
        CompInfo(i,2) = 0; %false does not match
    end

    %end
end
% 
%     %coder.varsize('CompBoundries',[960 1280], [1 0]);
% for k = 1 : CompNum           % Loop through all comp.
%     % Place the comp label number at the centroid of the blob.
%     if(CompInfo(k,2)==1)
% %text(centroidsX(k), centroidsY(k), num2str(k), 'FontSize', 14, 'FontWeight', 'Bold', 'HorizontalAlignment', 'center', 'VerticalAlignment', 'middle');
%     CompBoundries = bwboundaries(ConnComp,8,'noholes');
%     hold on;
%     thisBoundary = CompBoundries{k}; % Get boundary for this component
% 
%     InitBoundaryCoords(:,1,k) = thisBoundary(:,1);
%     InitBoundaryCoords(:,2,k) = thisBoundary(:,2);
%     % Column 2 is the columns, which is x % Column 1 is the rows, which is y
%     %plot(x, y, 'r-', 'LineWidth', 3.5); % Plot boundary in red.
%     end
% end

== matlab function IGVC2023_LaneLines_PublishingwLabels/MATLAB Function7 ==
  data: im input; results output uint8; imTest input; EnableTest input
function results = myimselect(im, imTest,EnableTest)
%Image Processing Function
%
% IM      - Input image.
% RESULTS - A scalar structure with the processing results.
%

%--------------------------------------------------------------------------
% Auto-generated by imageBatchProcessor App. 
%
% When used by the App, this function will be called for every input image
% file automatically. IM contains the input image as a matrix. RESULTS is a
% scalar structure containing the results of this processing function.
%
%--------------------------------------------------------------------------


persistent imageWork

if isempty(imageWork)
    imageWork=uint8(zeros(960,1280,3));
end

results=imageWork;

% Replace the sample below with your code----------------------------------

if EnableTest==1
    results=imTest;
else
    results=im;
end

%--------------------------------------------------------------------------

== matlab function IGVC2023_LaneLines_PublishingwLabels/ApplyROI ==
  data: RoiImg output; ImageOut input
function RoiImg = fcn(ImageOut)

RoiImg = ImageOut;
RoiImg(1:350,:,:)=0;

% function [ImageCrapped, sizeImage] = cropImage(ImageIn)
% 
% ImageCrapped = ImageIn;
% 
% ImageCrapped(1:410,:,:) = 0;
% 
% sizeImage = size(ImageCrapped);

== matlab function IGVC2023_LaneLines_PublishingwLabels/Filter Components  ==
  data: BW input; BWfiltered output
function BWfiltered = fcn(BW)

BWfiltered = bwareaopen(BW , 800);
